simulink model "LAB1_Unipolar Polar"  (R2020a)
settings: Solver=VariableStepAuto  StartTime=0.0  StopTime=10.0  RelTol=1e-3
libraries: commrandsrc3 x1
settings Model: Creator=Sameer  LastModifiedBy=Sameer

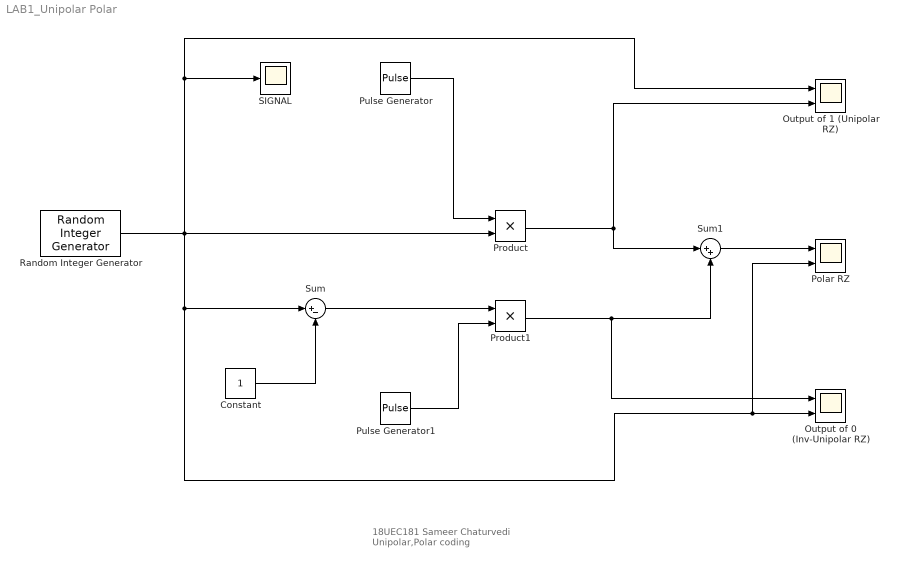
== system LAB1_Unipolar Polar ==
  note: 18UEC181
      | Sameer Chaturvedi
      | Unipolar,Polar coding
  Constant : Constant
  Output of 0 (Inv-Unipolar RZ) : Scope  NumInputPorts=2
  Output of 1 (Unipolar RZ) : Scope  NumInputPorts=2
  Polar RZ : Scope  NumInputPorts=2
  Product : Product
  Product1 : Product
  Pulse Generator : DiscretePulseGenerator  PulseType=Time based  Period=1  PulseWidth=50
  Pulse Generator1 : DiscretePulseGenerator  PulseType=Time based  Period=1  PulseWidth=50
  Random Integer Generator : commrandsrc3/Random Integer Generator  SetSize=2  SeedSource=Auto  Seed=0  SampleTime=1  SamplesPerFrame=1  OutputDataType=double  SimulateUsing=Interpreted execution
  SIGNAL : Scope
      settings: Description=SIGNAL
  Sum : Sum  Inputs=|+-
  Sum1 : Sum  Inputs=|++
  wires:
  Constant/1 -> Sum/2
  Random Integer Generator/1 -> Product/2, SIGNAL/1, Output of 1 (Unipolar RZ)/1, Polar RZ/2, Output of 0 (Inv-Unipolar RZ)/2, Sum/1
  Pulse Generator/1 -> Product/1
  Sum/1 -> Product1/1
  Pulse Generator1/1 -> Product1/2
  Product1/1 -> Output of 0 (Inv-Unipolar RZ)/1, Sum1/2
  Product/1 -> Sum1/1, Output of 1 (Unipolar RZ)/2
  Sum1/1 -> Polar RZ/1
